simulink model "msdft_12_v2"  (R2013b)
settings: Solver=ode45  StartTime=0.0  StopTime=10.0  RelTol=1e-3
undefined symbols (not defined in the file or in its folder): msdft, sys_lib
libraries: xbsIndex_r4 x3195, casper_library_misc x152, casper_library_delays x42, dspsigops x32, xps_library x3
(part 4 of 33)

== system msdft_12_v2/corr3 ==
  addr : Inport
  data_in : Inport  Port=2
  we : Inport  Port=3
  calc_add : Subsystem  mask{data_width=128, addr_width=10, sample_rate=sample_rate}
      mask prompts: data_width "data width"; addr_width "address width"; sample_rate "sample rate"
  convert_addr : xbsIndex_r4/Convert  gui_display_data_type=Fixed-point  arith_type=Unsigned  n_bits=addr_width  bin_pt=0  float_type=Single  exp_bits=8  fraction_bits=24  quantization=Truncate  overflow=Wrap  en=off  latency=0  dbl_ovrd=off  pipeline=off  block_type=convert
      settings: xl_area=[0, 0, 0, 0, 0, 0, 0]
  convert_din1 : xbsIndex_r4/Convert  gui_display_data_type=Fixed-point  arith_type=Unsigned  n_bits=128  bin_pt=0  float_type=Single  exp_bits=8  fraction_bits=24  quantization=Truncate  overflow=Wrap  en=off  latency=0  dbl_ovrd=off  pipeline=off  block_type=convert
      settings: xl_area=[0, 0, 0, 0, 0, 0, 0]
  convert_we : xbsIndex_r4/Convert  gui_display_data_type=Fixed-point  arith_type=Unsigned  n_bits=1  bin_pt=0  float_type=Single  exp_bits=8  fraction_bits=24  quantization=Truncate  overflow=Wrap  en=off  latency=0  dbl_ovrd=off  pipeline=off  block_type=convert
      settings: xl_area=[0, 0, 0, 0, 0, 0, 0]
  mem : Subsystem
  msdft_12_v2_corr3_addr : xbsIndex_r4/Gateway Out  inherit_from_input=off  hdl_port=on  timing_constraint=None  locs_specified=off  LOCs={'A5','B9','A9','C1','A3','G6','E9','A6','A7','A8','B8','B1','B3','D9','B5','B4','B6','C2'}  UseAsDAC=off  DACChannel='1'  block_type=gatewayout
      settings: infoedit="Gateway out block.  Converts Xilinx fixed point inputs into ouputs of type Simulink integer, double, or fixed point.<P><P>Hardware notes:  In hardware these blocks become top level output ports or are discarded, depending on how they are configured."  xl_area=[0, 0, 0, 0, 0, 0, 0]  sginterface={'Nallatech'=>{'xdspkit'=>{'non_memory_mapped_port'=>'uprev_Shared_BRAM_addr'}},'Xilinx'=>{'jtaghwcosim'=>{'non_memory_mapped_port'=>'uprev_Shared_BRAM_addr'},'xdspkit'=>{'non_memory_mapped_port'=>'uprev_Shared_BRAM_addr'}}}
  msdft_12_v2_corr3_data_in : xbsIndex_r4/Gateway Out  inherit_from_input=off  hdl_port=on  timing_constraint=None  locs_specified=off  LOCs={'B21','B22','A22','B23','B19','C19','A20','A21','A23','B24','A24','A25','E18','D18','C18','B18'}  UseAsDAC=off  DACChannel='1'  block_type=gatewayout
      settings: infoedit="Gateway out block.  Converts Xilinx fixed point inputs into ouputs of type Simulink integer, double, or fixed point.<P><P>Hardware notes:  In hardware these blocks become top level output ports or are discarded, depending on how they are configured."  xl_area=[0, 0, 0, 0, 0, 0, 0]  sginterface={'Nallatech'=>{'xdspkit'=>{'non_memory_mapped_port'=>'uprev_Shared_BRAM_data_in'}},'Xilinx'=>{'jtaghwcosim'=>{'non_memory_mapped_port'=>'uprev_Shared_BRAM_data_in'},'xdspkit'=>{'non_memory_mapped_port'=>'uprev_Shared_BRAM_data_in'}}}
  msdft_12_v2_corr3_data_out : xbsIndex_r4/Gateway In  gui_display_data_type=Fixed-point  arith_type=Unsigned  n_bits=128  bin_pt=0  preci_type=Single  exp_width=8  frac_width=24  quantization=Truncate  overflow=Wrap  period=sample_rate  dbl_ovrd=off  timing_constraint=None  locs_specified=off  LOCs={}  UseAsADC=off  ADCChannel='1'  inherit_from_input=off  hdl_port=on  block_type=gatewayin
      settings: xl_area=[0, 0, 0, 0, 0, 0, 0]
  msdft_12_v2_corr3_we : xbsIndex_r4/Gateway Out  inherit_from_input=off  hdl_port=on  timing_constraint=None  locs_specified=off  LOCs={'A14'}  UseAsDAC=off  DACChannel='1'  block_type=gatewayout
      settings: infoedit="Gateway out block.  Converts Xilinx fixed point inputs into ouputs of type Simulink integer, double, or fixed point.<P><P>Hardware notes:  In hardware these blocks become top level output ports or are discarded, depending on how they are configured."  xl_area=[0, 0, 0, 0, 0, 0, 0]
  munge_in : Subsystem  AncestorBlock=casper_library_flow_control/munge  mask(munge){divisions=4, div_size=[32 32 32 32], order=[3  2  1  0], arith_type_out=Unsigned, bin_pt_out=0}
      mask prompts: divisions "Number of divisions"; div_size "Division size (bits)"; order "Division packing order"; arith_type_out "Output arithmetic type"; bin_pt_out "Output binary point"
      mask help: Splits an input bus into the specified number of divisions and then recombines them in the order specified (most significant division = 0,least = number divisions-1)
      mask init:
      | munge_init(gcb, ...
      |     'divisions', divisions, ...
      |     'div_size', div_size, ...
      |     'order', order, ...
      |     'arith_type_out', arith_type_out, ...
      |     'bin_pt_out', bin_pt_out);
      settings: AttributesFormatString=|
      | split:[32 32 32 32]
      | join:[3 2 1 0]
      | Unsigned [128,0]
      mask TypeOptions arith_type_out: Unsigned | Signed  (2's comp) | Floating-point
  munge_out : Subsystem  AncestorBlock=casper_library_flow_control/munge  mask(munge){divisions=4, div_size=[32 32 32 32], order=[3  2  1  0], arith_type_out=Unsigned, bin_pt_out=0}
      mask prompts: divisions "Number of divisions"; div_size "Division size (bits)"; order "Division packing order"; arith_type_out "Output arithmetic type"; bin_pt_out "Output binary point"
      mask help: Splits an input bus into the specified number of divisions and then recombines them in the order specified (most significant division = 0,least = number divisions-1)
      mask init:
      | munge_init(gcb, ...
      |     'divisions', divisions, ...
      |     'div_size', div_size, ...
      |     'order', order, ...
      |     'arith_type_out', arith_type_out, ...
      |     'bin_pt_out', bin_pt_out);
      settings: AttributesFormatString=|
      | split:[32 32 32 32]
      | join:[3 2 1 0]
      | Unsigned [128,0]
      mask TypeOptions arith_type_out: Unsigned | Signed  (2's comp) | Floating-point
  data_out : Outport
  wires:
  convert_addr/1 -> msdft_12_v2_corr3_addr/1
  convert_din1/1 -> msdft_12_v2_corr3_data_in/1
  data_in/1 -> munge_in/1(din)
  calc_add/1(out) -> convert_addr/1
  msdft_12_v2_corr3_we/1 -> mem/3(In3)
  msdft_12_v2_corr3_data_in/1 -> mem/2(In2)
  msdft_12_v2_corr3_addr/1 -> mem/1(In1)
  convert_we/1 -> msdft_12_v2_corr3_we/1
  msdft_12_v2_corr3_data_out/1 -> munge_out/1(din)
  mem/1(Out1) -> msdft_12_v2_corr3_data_out/1
  addr/1 -> calc_add/1(in)
  we/1 -> convert_we/1
  munge_out/1(dout) -> data_out/1
  munge_in/1(dout) -> convert_din1/1

== system msdft_12_v2/corr4 ==
  addr : Inport
  data_in : Inport  Port=2
  we : Inport  Port=3
  calc_add : Subsystem  mask{data_width=128, addr_width=10, sample_rate=sample_rate}
      mask prompts: data_width "data width"; addr_width "address width"; sample_rate "sample rate"
  convert_addr : xbsIndex_r4/Convert  gui_display_data_type=Fixed-point  arith_type=Unsigned  n_bits=addr_width  bin_pt=0  float_type=Single  exp_bits=8  fraction_bits=24  quantization=Truncate  overflow=Wrap  en=off  latency=0  dbl_ovrd=off  pipeline=off  block_type=convert
      settings: xl_area=[0, 0, 0, 0, 0, 0, 0]
  convert_din1 : xbsIndex_r4/Convert  gui_display_data_type=Fixed-point  arith_type=Unsigned  n_bits=128  bin_pt=0  float_type=Single  exp_bits=8  fraction_bits=24  quantization=Truncate  overflow=Wrap  en=off  latency=0  dbl_ovrd=off  pipeline=off  block_type=convert
      settings: xl_area=[0, 0, 0, 0, 0, 0, 0]
  convert_we : xbsIndex_r4/Convert  gui_display_data_type=Fixed-point  arith_type=Unsigned  n_bits=1  bin_pt=0  float_type=Single  exp_bits=8  fraction_bits=24  quantization=Truncate  overflow=Wrap  en=off  latency=0  dbl_ovrd=off  pipeline=off  block_type=convert
      settings: xl_area=[0, 0, 0, 0, 0, 0, 0]
  mem : Subsystem
  msdft_12_v2_corr4_addr : xbsIndex_r4/Gateway Out  inherit_from_input=off  hdl_port=on  timing_constraint=None  locs_specified=off  LOCs={'A5','B9','A9','C1','A3','G6','E9','A6','A7','A8','B8','B1','B3','D9','B5','B4','B6','C2'}  UseAsDAC=off  DACChannel='1'  block_type=gatewayout
      settings: infoedit="Gateway out block.  Converts Xilinx fixed point inputs into ouputs of type Simulink integer, double, or fixed point.<P><P>Hardware notes:  In hardware these blocks become top level output ports or are discarded, depending on how they are configured."  xl_area=[0, 0, 0, 0, 0, 0, 0]  sginterface={'Nallatech'=>{'xdspkit'=>{'non_memory_mapped_port'=>'uprev_Shared_BRAM_addr'}},'Xilinx'=>{'jtaghwcosim'=>{'non_memory_mapped_port'=>'uprev_Shared_BRAM_addr'},'xdspkit'=>{'non_memory_mapped_port'=>'uprev_Shared_BRAM_addr'}}}
  msdft_12_v2_corr4_data_in : xbsIndex_r4/Gateway Out  inherit_from_input=off  hdl_port=on  timing_constraint=None  locs_specified=off  LOCs={'B21','B22','A22','B23','B19','C19','A20','A21','A23','B24','A24','A25','E18','D18','C18','B18'}  UseAsDAC=off  DACChannel='1'  block_type=gatewayout
      settings: infoedit="Gateway out block.  Converts Xilinx fixed point inputs into ouputs of type Simulink integer, double, or fixed point.<P><P>Hardware notes:  In hardware these blocks become top level output ports or are discarded, depending on how they are configured."  xl_area=[0, 0, 0, 0, 0, 0, 0]  sginterface={'Nallatech'=>{'xdspkit'=>{'non_memory_mapped_port'=>'uprev_Shared_BRAM_data_in'}},'Xilinx'=>{'jtaghwcosim'=>{'non_memory_mapped_port'=>'uprev_Shared_BRAM_data_in'},'xdspkit'=>{'non_memory_mapped_port'=>'uprev_Shared_BRAM_data_in'}}}
  msdft_12_v2_corr4_data_out : xbsIndex_r4/Gateway In  gui_display_data_type=Fixed-point  arith_type=Unsigned  n_bits=128  bin_pt=0  preci_type=Single  exp_width=8  frac_width=24  quantization=Truncate  overflow=Wrap  period=sample_rate  dbl_ovrd=off  timing_constraint=None  locs_specified=off  LOCs={}  UseAsADC=off  ADCChannel='1'  inherit_from_input=off  hdl_port=on  block_type=gatewayin
      settings: xl_area=[0, 0, 0, 0, 0, 0, 0]
  msdft_12_v2_corr4_we : xbsIndex_r4/Gateway Out  inherit_from_input=off  hdl_port=on  timing_constraint=None  locs_specified=off  LOCs={'A14'}  UseAsDAC=off  DACChannel='1'  block_type=gatewayout
      settings: infoedit="Gateway out block.  Converts Xilinx fixed point inputs into ouputs of type Simulink integer, double, or fixed point.<P><P>Hardware notes:  In hardware these blocks become top level output ports or are discarded, depending on how they are configured."  xl_area=[0, 0, 0, 0, 0, 0, 0]
  munge_in : Subsystem  AncestorBlock=casper_library_flow_control/munge  mask(munge){divisions=4, div_size=[32 32 32 32], order=[3  2  1  0], arith_type_out=Unsigned, bin_pt_out=0}
      mask prompts: divisions "Number of divisions"; div_size "Division size (bits)"; order "Division packing order"; arith_type_out "Output arithmetic type"; bin_pt_out "Output binary point"
      mask help: Splits an input bus into the specified number of divisions and then recombines them in the order specified (most significant division = 0,least = number divisions-1)
      mask init:
      | munge_init(gcb, ...
      |     'divisions', divisions, ...
      |     'div_size', div_size, ...
      |     'order', order, ...
      |     'arith_type_out', arith_type_out, ...
      |     'bin_pt_out', bin_pt_out);
      settings: AttributesFormatString=|
      | split:[32 32 32 32]
      | join:[3 2 1 0]
      | Unsigned [128,0]
      mask TypeOptions arith_type_out: Unsigned | Signed  (2's comp) | Floating-point
  munge_out : Subsystem  AncestorBlock=casper_library_flow_control/munge  mask(munge){divisions=4, div_size=[32 32 32 32], order=[3  2  1  0], arith_type_out=Unsigned, bin_pt_out=0}
      mask prompts: divisions "Number of divisions"; div_size "Division size (bits)"; order "Division packing order"; arith_type_out "Output arithmetic type"; bin_pt_out "Output binary point"
      mask help: Splits an input bus into the specified number of divisions and then recombines them in the order specified (most significant division = 0,least = number divisions-1)
      mask init:
      | munge_init(gcb, ...
      |     'divisions', divisions, ...
      |     'div_size', div_size, ...
      |     'order', order, ...
      |     'arith_type_out', arith_type_out, ...
      |     'bin_pt_out', bin_pt_out);
      settings: AttributesFormatString=|
      | split:[32 32 32 32]
      | join:[3 2 1 0]
      | Unsigned [128,0]
      mask TypeOptions arith_type_out: Unsigned | Signed  (2's comp) | Floating-point
  data_out : Outport
  wires:
  convert_addr/1 -> msdft_12_v2_corr4_addr/1
  convert_din1/1 -> msdft_12_v2_corr4_data_in/1
  data_in/1 -> munge_in/1(din)
  calc_add/1(out) -> convert_addr/1
  msdft_12_v2_corr4_we/1 -> mem/3(In3)
  msdft_12_v2_corr4_data_in/1 -> mem/2(In2)
  msdft_12_v2_corr4_addr/1 -> mem/1(In1)
  convert_we/1 -> msdft_12_v2_corr4_we/1
  msdft_12_v2_corr4_data_out/1 -> munge_out/1(din)
  mem/1(Out1) -> msdft_12_v2_corr4_data_out/1
  addr/1 -> calc_add/1(in)
  we/1 -> convert_we/1
  munge_out/1(dout) -> data_out/1
  munge_in/1(dout) -> convert_din1/1

== system msdft_12_v2/corr5 ==
  addr : Inport
  data_in : Inport  Port=2
  we : Inport  Port=3
  calc_add : Subsystem  mask{data_width=128, addr_width=10, sample_rate=sample_rate}
      mask prompts: data_width "data width"; addr_width "address width"; sample_rate "sample rate"
  convert_addr : xbsIndex_r4/Convert  gui_display_data_type=Fixed-point  arith_type=Unsigned  n_bits=addr_width  bin_pt=0  float_type=Single  exp_bits=8  fraction_bits=24  quantization=Truncate  overflow=Wrap  en=off  latency=0  dbl_ovrd=off  pipeline=off  block_type=convert
      settings: xl_area=[0, 0, 0, 0, 0, 0, 0]
  convert_din1 : xbsIndex_r4/Convert  gui_display_data_type=Fixed-point  arith_type=Unsigned  n_bits=128  bin_pt=0  float_type=Single  exp_bits=8  fraction_bits=24  quantization=Truncate  overflow=Wrap  en=off  latency=0  dbl_ovrd=off  pipeline=off  block_type=convert
      settings: xl_area=[0, 0, 0, 0, 0, 0, 0]
  convert_we : xbsIndex_r4/Convert  gui_display_data_type=Fixed-point  arith_type=Unsigned  n_bits=1  bin_pt=0  float_type=Single  exp_bits=8  fraction_bits=24  quantization=Truncate  overflow=Wrap  en=off  latency=0  dbl_ovrd=off  pipeline=off  block_type=convert
      settings: xl_area=[0, 0, 0, 0, 0, 0, 0]
  mem : Subsystem
  msdft_12_v2_corr5_addr : xbsIndex_r4/Gateway Out  inherit_from_input=off  hdl_port=on  timing_constraint=None  locs_specified=off  LOCs={'A5','B9','A9','C1','A3','G6','E9','A6','A7','A8','B8','B1','B3','D9','B5','B4','B6','C2'}  UseAsDAC=off  DACChannel='1'  block_type=gatewayout
      settings: infoedit="Gateway out block.  Converts Xilinx fixed point inputs into ouputs of type Simulink integer, double, or fixed point.<P><P>Hardware notes:  In hardware these blocks become top level output ports or are discarded, depending on how they are configured."  xl_area=[0, 0, 0, 0, 0, 0, 0]  sginterface={'Nallatech'=>{'xdspkit'=>{'non_memory_mapped_port'=>'uprev_Shared_BRAM_addr'}},'Xilinx'=>{'jtaghwcosim'=>{'non_memory_mapped_port'=>'uprev_Shared_BRAM_addr'},'xdspkit'=>{'non_memory_mapped_port'=>'uprev_Shared_BRAM_addr'}}}
  msdft_12_v2_corr5_data_in : xbsIndex_r4/Gateway Out  inherit_from_input=off  hdl_port=on  timing_constraint=None  locs_specified=off  LOCs={'B21','B22','A22','B23','B19','C19','A20','A21','A23','B24','A24','A25','E18','D18','C18','B18'}  UseAsDAC=off  DACChannel='1'  block_type=gatewayout
      settings: infoedit="Gateway out block.  Converts Xilinx fixed point inputs into ouputs of type Simulink integer, double, or fixed point.<P><P>Hardware notes:  In hardware these blocks become top level output ports or are discarded, depending on how they are configured."  xl_area=[0, 0, 0, 0, 0, 0, 0]  sginterface={'Nallatech'=>{'xdspkit'=>{'non_memory_mapped_port'=>'uprev_Shared_BRAM_data_in'}},'Xilinx'=>{'jtaghwcosim'=>{'non_memory_mapped_port'=>'uprev_Shared_BRAM_data_in'},'xdspkit'=>{'non_memory_mapped_port'=>'uprev_Shared_BRAM_data_in'}}}
  msdft_12_v2_corr5_data_out : xbsIndex_r4/Gateway In  gui_display_data_type=Fixed-point  arith_type=Unsigned  n_bits=128  bin_pt=0  preci_type=Single  exp_width=8  frac_width=24  quantization=Truncate  overflow=Wrap  period=sample_rate  dbl_ovrd=off  timing_constraint=None  locs_specified=off  LOCs={}  UseAsADC=off  ADCChannel='1'  inherit_from_input=off  hdl_port=on  block_type=gatewayin
      settings: xl_area=[0, 0, 0, 0, 0, 0, 0]
  msdft_12_v2_corr5_we : xbsIndex_r4/Gateway Out  inherit_from_input=off  hdl_port=on  timing_constraint=None  locs_specified=off  LOCs={'A14'}  UseAsDAC=off  DACChannel='1'  block_type=gatewayout
      settings: infoedit="Gateway out block.  Converts Xilinx fixed point inputs into ouputs of type Simulink integer, double, or fixed point.<P><P>Hardware notes:  In hardware these blocks become top level output ports or are discarded, depending on how they are configured."  xl_area=[0, 0, 0, 0, 0, 0, 0]
  munge_in : Subsystem  AncestorBlock=casper_library_flow_control/munge  mask(munge){divisions=4, div_size=[32 32 32 32], order=[3  2  1  0], arith_type_out=Unsigned, bin_pt_out=0}
      mask prompts: divisions "Number of divisions"; div_size "Division size (bits)"; order "Division packing order"; arith_type_out "Output arithmetic type"; bin_pt_out "Output binary point"
      mask help: Splits an input bus into the specified number of divisions and then recombines them in the order specified (most significant division = 0,least = number divisions-1)
      mask init:
      | munge_init(gcb, ...
      |     'divisions', divisions, ...
      |     'div_size', div_size, ...
      |     'order', order, ...
      |     'arith_type_out', arith_type_out, ...
      |     'bin_pt_out', bin_pt_out);
      settings: AttributesFormatString=|
      | split:[32 32 32 32]
      | join:[3 2 1 0]
      | Unsigned [128,0]
      mask TypeOptions arith_type_out: Unsigned | Signed  (2's comp) | Floating-point
  munge_out : Subsystem  AncestorBlock=casper_library_flow_control/munge  mask(munge){divisions=4, div_size=[32 32 32 32], order=[3  2  1  0], arith_type_out=Unsigned, bin_pt_out=0}
      mask prompts: divisions "Number of divisions"; div_size "Division size (bits)"; order "Division packing order"; arith_type_out "Output arithmetic type"; bin_pt_out "Output binary point"
      mask help: Splits an input bus into the specified number of divisions and then recombines them in the order specified (most significant division = 0,least = number divisions-1)
      mask init:
      | munge_init(gcb, ...
      |     'divisions', divisions, ...
      |     'div_size', div_size, ...
      |     'order', order, ...
      |     'arith_type_out', arith_type_out, ...
      |     'bin_pt_out', bin_pt_out);
      settings: AttributesFormatString=|
      | split:[32 32 32 32]
      | join:[3 2 1 0]
      | Unsigned [128,0]
      mask TypeOptions arith_type_out: Unsigned | Signed  (2's comp) | Floating-point
  data_out : Outport
  wires:
  convert_addr/1 -> msdft_12_v2_corr5_addr/1
  convert_din1/1 -> msdft_12_v2_corr5_data_in/1
  data_in/1 -> munge_in/1(din)
  calc_add/1(out) -> convert_addr/1
  msdft_12_v2_corr5_we/1 -> mem/3(In3)
  msdft_12_v2_corr5_data_in/1 -> mem/2(In2)
  msdft_12_v2_corr5_addr/1 -> mem/1(In1)
  convert_we/1 -> msdft_12_v2_corr5_we/1
  msdft_12_v2_corr5_data_out/1 -> munge_out/1(din)
  mem/1(Out1) -> msdft_12_v2_corr5_data_out/1
  addr/1 -> calc_add/1(in)
  we/1 -> convert_we/1
  munge_out/1(dout) -> data_out/1
  munge_in/1(dout) -> convert_din1/1

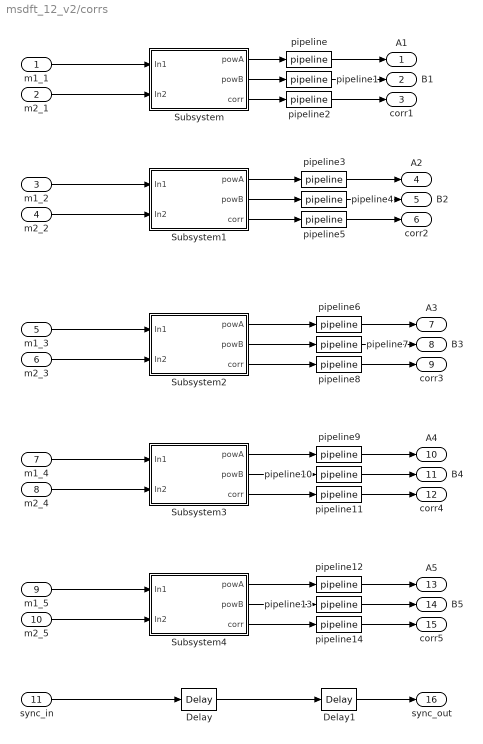
== system msdft_12_v2/corrs ==
  m1_1 : Inport
  m2_1 : Inport  Port=2
  m1_2 : Inport  Port=3
  m2_2 : Inport  Port=4
  m1_3 : Inport  Port=5
  m2_3 : Inport  Port=6
  m1_4 : Inport  Port=7
  m2_4 : Inport  Port=8
  m1_5 : Inport  Port=9
  m2_5 : Inport  Port=10
  sync_in : Inport  Port=11
  Delay : xbsIndex_r4/Delay  rst=off  infoeditControl=Selection of Reset will increase slice count due to use of real FFs and instead of SRLs  en=off  latency=10  dbl_ovrd=off  reg_retiming=off  block_type=delay
  Delay1 : xbsIndex_r4/Delay  rst=off  infoeditControl=Selection of Reset will increase slice count due to use of real FFs and instead of SRLs  en=off  latency=3  dbl_ovrd=off  reg_retiming=off  block_type=delay
  Subsystem : Subsystem
  Subsystem1 : Subsystem
  Subsystem2 : Subsystem
  Subsystem3 : Subsystem
  Subsystem4 : Subsystem
  pipeline{,1..14} (15 alike) : casper_library_delays/pipeline  latency=3
      settings: AttributesFormatString=Latency = %<latency>
  A1 : Outport
  B1 : Outport  Port=2
  corr1 : Outport  Port=3
  A2 : Outport  Port=4
  B2 : Outport  Port=5
  corr2 : Outport  Port=6
  A3 : Outport  Port=7
  B3 : Outport  Port=8
  corr3 : Outport  Port=9
  A4 : Outport  Port=10
  B4 : Outport  Port=11
  corr4 : Outport  Port=12
  A5 : Outport  Port=13
  B5 : Outport  Port=14
  corr5 : Outport  Port=15
  sync_out : Outport  Port=16
  wires:
  m1_1/1 -> Subsystem/1(In1)
  m2_1/1 -> Subsystem/2(In2)
  m1_2/1 -> Subsystem1/1(In1)
  m2_2/1 -> Subsystem1/2(In2)
  m1_3/1 -> Subsystem2/1(In1)
  m2_3/1 -> Subsystem2/2(In2)
  m1_4/1 -> Subsystem3/1(In1)
  m2_4/1 -> Subsystem3/2(In2)
  m1_5/1 -> Subsystem4/1(In1)
  m2_5/1 -> Subsystem4/2(In2)
  Subsystem/1(powA) -> pipeline/1
  Subsystem/2(powB) -> pipeline1/1
  Subsystem/3(corr) -> pipeline2/1
  pipeline/1 -> A1/1
  pipeline1/1 -> B1/1
  pipeline2/1 -> corr1/1
  pipeline3/1 -> A2/1
  pipeline4/1 -> B2/1
  pipeline5/1 -> corr2/1
  Subsystem1/1(powA) -> pipeline3/1
  Subsystem1/2(powB) -> pipeline4/1
  Subsystem1/3(corr) -> pipeline5/1
  pipeline6/1 -> A3/1
  pipeline7/1 -> B3/1
  pipeline8/1 -> corr3/1
  Subsystem2/1(powA) -> pipeline6/1
  Subsystem2/2(powB) -> pipeline7/1
  Subsystem2/3(corr) -> pipeline8/1
  pipeline9/1 -> A4/1
  pipeline10/1 -> B4/1
  pipeline11/1 -> corr4/1
  Subsystem3/1(powA) -> pipeline9/1
  Subsystem3/2(powB) -> pipeline10/1
  Subsystem3/3(corr) -> pipeline11/1
  pipeline12/1 -> A5/1
  pipeline13/1 -> B5/1
  pipeline14/1 -> corr5/1
  Subsystem4/1(powA) -> pipeline12/1
  Subsystem4/2(powB) -> pipeline13/1
  Subsystem4/3(corr) -> pipeline14/1
  sync_in/1 -> Delay/1
  Delay/1 -> Delay1/1
  Delay1/1 -> sync_out/1

== system msdft_12_v2/mem_addr ==
  sim_1 : Inport
  io_delay : xbsIndex_r4/Delay  rst=off  infoeditControl=Selection of Reset will increase slice count due to use of real FFs and instead of SRLs  en=off  latency=0  dbl_ovrd=off  reg_retiming=on  block_type=delay
  msdft_12_v2_mem_addr_user_data_out : xbsIndex_r4/Gateway In  gui_display_data_type=Fixed-point  arith_type=Unsigned  n_bits=32  bin_pt=0  preci_type=Single  exp_width=8  frac_width=24  quantization="Round  (unbiased: +/- Inf)"  overflow=Saturate  period=1  dbl_ovrd=off  timing_constraint=None  locs_specified=off  LOCs={}  UseAsADC=off  ADCChannel='1'  inherit_from_input=off  hdl_port=on  block_type=gatewayin
  reint1 : xbsIndex_r4/Reinterpret  force_arith_type=on  arith_type=Unsigned  force_bin_pt=on  bin_pt=0  block_type=reinterpret
  slice_reg : xbsIndex_r4/Slice  nbits=32  boolean_output=off  mode=Lower Bit Location + Width  bit1=0  base1=MSB of Input  bit0=0  base0=LSB of Input  dbl_ovrd=off  block_type=slice
  in_reg : Outport
  wires:
  msdft_12_v2_mem_addr_user_data_out/1 -> io_delay/1
  sim_1/1 -> msdft_12_v2_mem_addr_user_data_out/1
  io_delay/1 -> slice_reg/1
  slice_reg/1 -> reint1/1
  reint1/1 -> in_reg/1

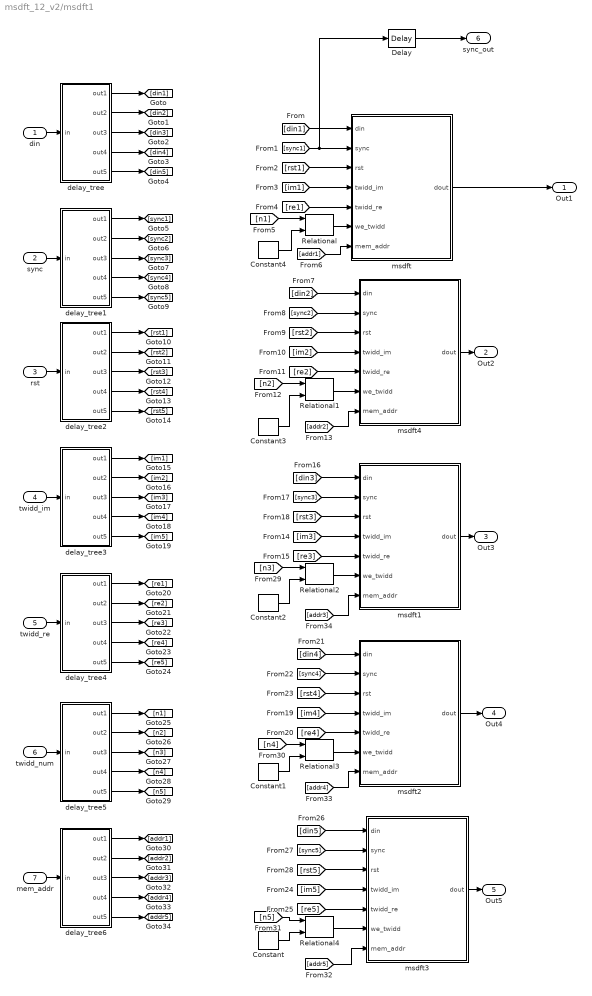
== system msdft_12_v2/msdft1 ==
  din : Inport
  "sync " : Inport  Port=2
  rst : Inport  Port=3
  twidd_im : Inport  Port=4
  twidd_re : Inport  Port=5
  twidd_num : Inport  Port=6
  mem_addr : Inport  Port=7
  Constant : xbsIndex_r4/Constant  const=5  gui_display_data_type=Fixed-point  arith_type=Unsigned  n_bits=16  bin_pt=0  preci_type=Single  exp_width=8  frac_width=24  explicit_period=on  period=1  equ=P=C  opselect=C  inp2=PCIN>>17  opr=+  inp1=P  carry=CIN  dbl_ovrd=off  block_type=constant
  Constant1 : xbsIndex_r4/Constant  const=4  gui_display_data_type=Fixed-point  arith_type=Unsigned  n_bits=16  bin_pt=0  preci_type=Single  exp_width=8  frac_width=24  explicit_period=on  period=1  equ=P=C  opselect=C  inp2=PCIN>>17  opr=+  inp1=P  carry=CIN  dbl_ovrd=off  block_type=constant
  Constant2 : xbsIndex_r4/Constant  const=3  gui_display_data_type=Fixed-point  arith_type=Unsigned  n_bits=16  bin_pt=0  preci_type=Single  exp_width=8  frac_width=24  explicit_period=on  period=1  equ=P=C  opselect=C  inp2=PCIN>>17  opr=+  inp1=P  carry=CIN  dbl_ovrd=off  block_type=constant
  Constant3 : xbsIndex_r4/Constant  const=2  gui_display_data_type=Fixed-point  arith_type=Unsigned  n_bits=16  bin_pt=0  preci_type=Single  exp_width=8  frac_width=24  explicit_period=on  period=1  equ=P=C  opselect=C  inp2=PCIN>>17  opr=+  inp1=P  carry=CIN  dbl_ovrd=off  block_type=constant
  Constant4 : xbsIndex_r4/Constant  const=1  gui_display_data_type=Fixed-point  arith_type=Unsigned  n_bits=16  bin_pt=0  preci_type=Single  exp_width=8  frac_width=24  explicit_period=on  period=1  equ=P=C  opselect=C  inp2=PCIN>>17  opr=+  inp1=P  carry=CIN  dbl_ovrd=off  block_type=constant
  Delay : xbsIndex_r4/Delay  rst=off  infoeditControl=Selection of Reset will increase slice count due to use of real FFs and instead of SRLs  en=off  latency=2^12+10  dbl_ovrd=off  reg_retiming=off  block_type=delay
  Relational{,1..4} (5 alike) : xbsIndex_r4/Relational  mode=a=b  en=off  latency=0  dbl_ovrd=off  block_type=relational
  delay_tree : Subsystem  AncestorBlock=casper_library_delays/delay_tree  mask(delay_tree){fanout=5, bfac=2}
      mask prompts: bfac "Branching factor"
      mask help: A tree of delays.
      mask init:
      | delay_tree_init(gcb, ...
      |     'fanout', fanout, ...
      |     'bfac', bfac);
      settings: AttributesFormatString=delay=4
  delay_tree1 : Subsystem  AncestorBlock=casper_library_delays/delay_tree  mask(delay_tree){fanout=5, bfac=2}
      mask prompts: bfac "Branching factor"
      mask help: A tree of delays.
      mask init:
      | delay_tree_init(gcb, ...
      |     'fanout', fanout, ...
      |     'bfac', bfac);
      settings: AttributesFormatString=delay=4
  delay_tree2 : Subsystem  AncestorBlock=casper_library_delays/delay_tree  mask(delay_tree){fanout=5, bfac=2}
      mask prompts: bfac "Branching factor"
      mask help: A tree of delays.
      mask init:
      | delay_tree_init(gcb, ...
      |     'fanout', fanout, ...
      |     'bfac', bfac);
      settings: AttributesFormatString=delay=4
  delay_tree3 : Subsystem  AncestorBlock=casper_library_delays/delay_tree  mask(delay_tree){fanout=5, bfac=2}
      mask prompts: bfac "Branching factor"
      mask help: A tree of delays.
      mask init:
      | delay_tree_init(gcb, ...
      |     'fanout', fanout, ...
      |     'bfac', bfac);
      settings: AttributesFormatString=delay=4
  delay_tree4 : Subsystem  AncestorBlock=casper_library_delays/delay_tree  mask(delay_tree){fanout=5, bfac=2}
      mask prompts: bfac "Branching factor"
      mask help: A tree of delays.
      mask init:
      | delay_tree_init(gcb, ...
      |     'fanout', fanout, ...
      |     'bfac', bfac);
      settings: AttributesFormatString=delay=4
  delay_tree5 : Subsystem  AncestorBlock=casper_library_delays/delay_tree  mask(delay_tree){fanout=5, bfac=2}
      mask prompts: bfac "Branching factor"
      mask help: A tree of delays.
      mask init:
      | delay_tree_init(gcb, ...
      |     'fanout', fanout, ...
      |     'bfac', bfac);
      settings: AttributesFormatString=delay=4
  delay_tree6 : Subsystem  AncestorBlock=casper_library_delays/delay_tree  mask(delay_tree){fanout=5, bfac=2}
      mask prompts: bfac "Branching factor"
      mask help: A tree of delays.
      mask init:
      | delay_tree_init(gcb, ...
      |     'fanout', fanout, ...
      |     'bfac', bfac);
      settings: AttributesFormatString=delay=4
  msdft : Subsystem  AncestorBlock=sys_lib/msdft  mask{in_bit=8, N=12, init_twidd=1397, twidd_bit=16, out_bit=25}
      mask prompts: in_bit "input bitwidth"; N "dft size (2^?)"; init_twidd "init twiddle factor"; twidd_bit "bitsize twiddle factor"; out_bit "output bitwidth"
  msdft1 : Subsystem  AncestorBlock=sys_lib/msdft  mask{in_bit=8, N=12, init_twidd=1399, twidd_bit=16, out_bit=25}
      mask prompts: in_bit "input bitwidth"; N "dft size (2^?)"; init_twidd "init twiddle factor"; twidd_bit "bitsize twiddle factor"; out_bit "output bitwidth"
  msdft2 : Subsystem  AncestorBlock=sys_lib/msdft  mask{in_bit=8, N=12, init_twidd=1400, twidd_bit=16, out_bit=25}
      mask prompts: in_bit "input bitwidth"; N "dft size (2^?)"; init_twidd "init twiddle factor"; twidd_bit "bitsize twiddle factor"; out_bit "output bitwidth"
  msdft3 : Subsystem  AncestorBlock=sys_lib/msdft  mask{in_bit=8, N=12, init_twidd=1401, twidd_bit=16, out_bit=25}
      mask prompts: in_bit "input bitwidth"; N "dft size (2^?)"; init_twidd "init twiddle factor"; twidd_bit "bitsize twiddle factor"; out_bit "output bitwidth"
  msdft4 : Subsystem  AncestorBlock=sys_lib/msdft  mask{in_bit=8, N=12, init_twidd=1398, twidd_bit=16, out_bit=25}
      mask prompts: in_bit "input bitwidth"; N "dft size (2^?)"; init_twidd "init twiddle factor"; twidd_bit "bitsize twiddle factor"; out_bit "output bitwidth"
  Out1 : Outport
  Out2 : Outport  Port=2
  Out3 : Outport  Port=3
  Out4 : Outport  Port=4
  Out5 : Outport  Port=5
  sync_out : Outport  Port=6
  wires:
  Constant3/1 -> Relational1/2
  [addr3] -> msdft1/7(mem_addr)
  [din5] -> msdft3/1(din)
  delay_tree6/1(out1) -> [addr1]
  Constant4/1 -> Relational/2
  msdft1/1(dout) -> Out3/1
  delay_tree6/3(out3) -> [addr3]
  [rst5] -> msdft3/3(rst)
  delay_tree5/4(out4) -> [n4]
  delay_tree5/5(out5) -> [n5]
  Constant2/1 -> Relational2/2
  delay_tree2/3(out3) -> [rst3]
  delay_tree4/1(out1) -> [re1]
  delay_tree3/4(out4) -> [im4]
  [rst1] -> msdft/3(rst)
  [re3] -> msdft1/5(twidd_re)
  [n3] -> Relational2/1
  delay_tree6/2(out2) -> [addr2]
  "sync "/1 -> delay_tree1/1(in)
  [addr5] -> msdft3/7(mem_addr)
  delay_tree/2(out2) -> [din2]
  delay_tree1/2(out2) -> [sync2]
  twidd_re/1 -> delay_tree4/1(in)
  delay_tree/3(out3) -> [din3]
  [din2] -> msdft4/1(din)
  Relational4/1 -> msdft3/6(we_twidd)
  [re5] -> msdft3/5(twidd_re)
  Relational1/1 -> msdft4/6(we_twidd)
  [re4] -> msdft2/5(twidd_re)
  delay_tree2/5(out5) -> [rst5]
  [sync4] -> msdft2/2(sync)
  delay_tree2/2(out2) -> [rst2]
  delay_tree/1(out1) -> [din1]
  [re2] -> msdft4/5(twidd_re)
  [sync1] -> Delay/1, msdft/2(sync)
  delay_tree4/3(out3) -> [re3]
  din/1 -> delay_tree/1(in)
  [sync5] -> msdft3/2(sync)
  [din4] -> msdft2/1(din)
  delay_tree3/1(out1) -> [im1]
  delay_tree1/4(out4) -> [sync4]
  delay_tree4/2(out2) -> [re2]
  [n5] -> Relational4/1
  delay_tree5/2(out2) -> [n2]
  [sync3] -> msdft1/2(sync)
  delay_tree1/5(out5) -> [sync5]
  delay_tree5/3(out3) -> [n3]
  [addr2] -> msdft4/7(mem_addr)
  [rst4] -> msdft2/3(rst)
  twidd_num/1 -> delay_tree5/1(in)
  Constant1/1 -> Relational3/2
  delay_tree5/1(out1) -> [n1]
  [din3] -> msdft1/1(din)
  rst/1 -> delay_tree2/1(in)
  msdft2/1(dout) -> Out4/1
  [addr1] -> msdft/7(mem_addr)
  [addr4] -> msdft2/7(mem_addr)
  delay_tree3/2(out2) -> [im2]
  delay_tree2/1(out1) -> [rst1]
  [im5] -> msdft3/4(twidd_im)
  delay_tree6/4(out4) -> [addr4]
  [n4] -> Relational3/1
  twidd_im/1 -> delay_tree3/1(in)
  [im1] -> msdft/4(twidd_im)
  delay_tree3/5(out5) -> [im5]
  msdft/1(dout) -> Out1/1
  [im4] -> msdft2/4(twidd_im)
  Relational/1 -> msdft/6(we_twidd)
  delay_tree3/3(out3) -> [im3]
  delay_tree2/4(out4) -> [rst4]
  [n2] -> Relational1/1
  [din1] -> msdft/1(din)
  delay_tree1/1(out1) -> [sync1]
  [im3] -> msdft1/4(twidd_im)
  Constant/1 -> Relational4/2
  delay_tree4/4(out4) -> [re4]
  [im2] -> msdft4/4(twidd_im)
  delay_tree4/5(out5) -> [re5]
  delay_tree6/5(out5) -> [addr5]
  delay_tree1/3(out3) -> [sync3]
  [rst3] -> msdft1/3(rst)
  [rst2] -> msdft4/3(rst)
  [n1] -> Relational/1
  Relational2/1 -> msdft1/6(we_twidd)
  [sync2] -> msdft4/2(sync)
  [re1] -> msdft/5(twidd_re)
  delay_tree/4(out4) -> [din4]
  Relational3/1 -> msdft2/6(we_twidd)
  mem_addr/1 -> delay_tree6/1(in)
  delay_tree/5(out5) -> [din5]
  Delay/1 -> sync_out/1
  msdft4/1(dout) -> Out2/1
  msdft3/1(dout) -> Out5/1

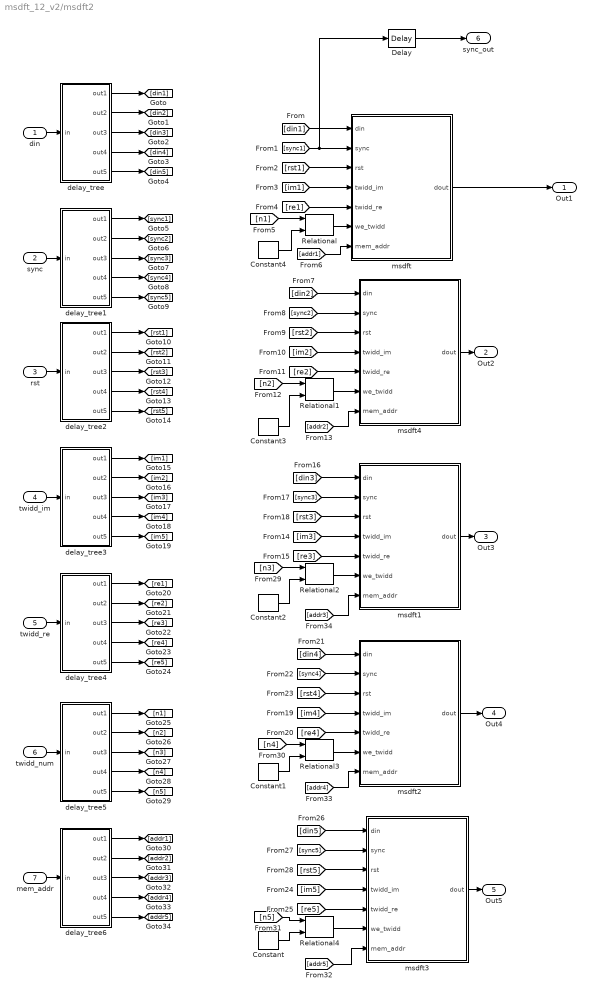
== system msdft_12_v2/msdft2 ==
  din : Inport
  "sync " : Inport  Port=2
  rst : Inport  Port=3
  twidd_im : Inport  Port=4
  twidd_re : Inport  Port=5
  twidd_num : Inport  Port=6
  mem_addr : Inport  Port=7
  Constant : xbsIndex_r4/Constant  const=5  gui_display_data_type=Fixed-point  arith_type=Unsigned  n_bits=16  bin_pt=0  preci_type=Single  exp_width=8  frac_width=24  explicit_period=on  period=1  equ=P=C  opselect=C  inp2=PCIN>>17  opr=+  inp1=P  carry=CIN  dbl_ovrd=off  block_type=constant
  Constant1 : xbsIndex_r4/Constant  const=4  gui_display_data_type=Fixed-point  arith_type=Unsigned  n_bits=16  bin_pt=0  preci_type=Single  exp_width=8  frac_width=24  explicit_period=on  period=1  equ=P=C  opselect=C  inp2=PCIN>>17  opr=+  inp1=P  carry=CIN  dbl_ovrd=off  block_type=constant
  Constant2 : xbsIndex_r4/Constant  const=3  gui_display_data_type=Fixed-point  arith_type=Unsigned  n_bits=16  bin_pt=0  preci_type=Single  exp_width=8  frac_width=24  explicit_period=on  period=1  equ=P=C  opselect=C  inp2=PCIN>>17  opr=+  inp1=P  carry=CIN  dbl_ovrd=off  block_type=constant
  Constant3 : xbsIndex_r4/Constant  const=2  gui_display_data_type=Fixed-point  arith_type=Unsigned  n_bits=16  bin_pt=0  preci_type=Single  exp_width=8  frac_width=24  explicit_period=on  period=1  equ=P=C  opselect=C  inp2=PCIN>>17  opr=+  inp1=P  carry=CIN  dbl_ovrd=off  block_type=constant
  Constant4 : xbsIndex_r4/Constant  const=1  gui_display_data_type=Fixed-point  arith_type=Unsigned  n_bits=16  bin_pt=0  preci_type=Single  exp_width=8  frac_width=24  explicit_period=on  period=1  equ=P=C  opselect=C  inp2=PCIN>>17  opr=+  inp1=P  carry=CIN  dbl_ovrd=off  block_type=constant
  Delay : xbsIndex_r4/Delay  rst=off  infoeditControl=Selection of Reset will increase slice count due to use of real FFs and instead of SRLs  en=off  latency=2^12+10  dbl_ovrd=off  reg_retiming=off  block_type=delay
  Relational{,1..4} (5 alike) : xbsIndex_r4/Relational  mode=a=b  en=off  latency=0  dbl_ovrd=off  block_type=relational
  delay_tree : Subsystem  AncestorBlock=casper_library_delays/delay_tree  mask(delay_tree){fanout=5, bfac=2}
      mask prompts: bfac "Branching factor"
      mask help: A tree of delays.
      mask init:
      | delay_tree_init(gcb, ...
      |     'fanout', fanout, ...
      |     'bfac', bfac);
      settings: AttributesFormatString=delay=4
  delay_tree1 : Subsystem  AncestorBlock=casper_library_delays/delay_tree  mask(delay_tree){fanout=5, bfac=2}
      mask prompts: bfac "Branching factor"
      mask help: A tree of delays.
      mask init:
      | delay_tree_init(gcb, ...
      |     'fanout', fanout, ...
      |     'bfac', bfac);
      settings: AttributesFormatString=delay=4
  delay_tree2 : Subsystem  AncestorBlock=casper_library_delays/delay_tree  mask(delay_tree){fanout=5, bfac=2}
      mask prompts: bfac "Branching factor"
      mask help: A tree of delays.
      mask init:
      | delay_tree_init(gcb, ...
      |     'fanout', fanout, ...
      |     'bfac', bfac);
      settings: AttributesFormatString=delay=4
  delay_tree3 : Subsystem  AncestorBlock=casper_library_delays/delay_tree  mask(delay_tree){fanout=5, bfac=2}
      mask prompts: bfac "Branching factor"
      mask help: A tree of delays.
      mask init:
      | delay_tree_init(gcb, ...
      |     'fanout', fanout, ...
      |     'bfac', bfac);
      settings: AttributesFormatString=delay=4
  delay_tree4 : Subsystem  AncestorBlock=casper_library_delays/delay_tree  mask(delay_tree){fanout=5, bfac=2}
      mask prompts: bfac "Branching factor"
      mask help: A tree of delays.
      mask init:
      | delay_tree_init(gcb, ...
      |     'fanout', fanout, ...
      |     'bfac', bfac);
      settings: AttributesFormatString=delay=4
  delay_tree5 : Subsystem  AncestorBlock=casper_library_delays/delay_tree  mask(delay_tree){fanout=5, bfac=2}
      mask prompts: bfac "Branching factor"
      mask help: A tree of delays.
      mask init:
      | delay_tree_init(gcb, ...
      |     'fanout', fanout, ...
      |     'bfac', bfac);
      settings: AttributesFormatString=delay=4
  delay_tree6 : Subsystem  AncestorBlock=casper_library_delays/delay_tree  mask(delay_tree){fanout=5, bfac=2}
      mask prompts: bfac "Branching factor"
      mask help: A tree of delays.
      mask init:
      | delay_tree_init(gcb, ...
      |     'fanout', fanout, ...
      |     'bfac', bfac);
      settings: AttributesFormatString=delay=4
  msdft : Subsystem  AncestorBlock=sys_lib/msdft  mask{in_bit=8, N=12, init_twidd=1397, twidd_bit=16, out_bit=25}
      mask prompts: in_bit "input bitwidth"; N "dft size (2^?)"; init_twidd "init twiddle factor"; twidd_bit "bitsize twiddle factor"; out_bit "output bitwidth"
  msdft1 : Subsystem  AncestorBlock=sys_lib/msdft  mask{in_bit=8, N=12, init_twidd=1399, twidd_bit=16, out_bit=25}
      mask prompts: in_bit "input bitwidth"; N "dft size (2^?)"; init_twidd "init twiddle factor"; twidd_bit "bitsize twiddle factor"; out_bit "output bitwidth"
  msdft2 : Subsystem  AncestorBlock=sys_lib/msdft  mask{in_bit=8, N=12, init_twidd=1400, twidd_bit=16, out_bit=25}
      mask prompts: in_bit "input bitwidth"; N "dft size (2^?)"; init_twidd "init twiddle factor"; twidd_bit "bitsize twiddle factor"; out_bit "output bitwidth"
  msdft3 : Subsystem  AncestorBlock=sys_lib/msdft  mask{in_bit=8, N=12, init_twidd=1401, twidd_bit=16, out_bit=25}
      mask prompts: in_bit "input bitwidth"; N "dft size (2^?)"; init_twidd "init twiddle factor"; twidd_bit "bitsize twiddle factor"; out_bit "output bitwidth"
  msdft4 : Subsystem  AncestorBlock=sys_lib/msdft  mask{in_bit=8, N=12, init_twidd=1398, twidd_bit=16, out_bit=25}
      mask prompts: in_bit "input bitwidth"; N "dft size (2^?)"; init_twidd "init twiddle factor"; twidd_bit "bitsize twiddle factor"; out_bit "output bitwidth"
  Out1 : Outport
  Out2 : Outport  Port=2
  Out3 : Outport  Port=3
  Out4 : Outport  Port=4
  Out5 : Outport  Port=5
  sync_out : Outport  Port=6
  wires:
  Constant3/1 -> Relational1/2
  [addr3] -> msdft1/7(mem_addr)
  [din5] -> msdft3/1(din)
  delay_tree6/1(out1) -> [addr1]
  Constant4/1 -> Relational/2
  msdft1/1(dout) -> Out3/1
  delay_tree6/3(out3) -> [addr3]
  [rst5] -> msdft3/3(rst)
  delay_tree5/4(out4) -> [n4]
  delay_tree5/5(out5) -> [n5]
  Constant2/1 -> Relational2/2
  delay_tree2/3(out3) -> [rst3]
  delay_tree4/1(out1) -> [re1]
  delay_tree3/4(out4) -> [im4]
  [rst1] -> msdft/3(rst)
  [re3] -> msdft1/5(twidd_re)
  [n3] -> Relational2/1
  delay_tree6/2(out2) -> [addr2]
  "sync "/1 -> delay_tree1/1(in)
  [addr5] -> msdft3/7(mem_addr)
  delay_tree/2(out2) -> [din2]
  delay_tree1/2(out2) -> [sync2]
  twidd_re/1 -> delay_tree4/1(in)
  delay_tree/3(out3) -> [din3]
  [din2] -> msdft4/1(din)
  Relational4/1 -> msdft3/6(we_twidd)
  [re5] -> msdft3/5(twidd_re)
  Relational1/1 -> msdft4/6(we_twidd)
  [re4] -> msdft2/5(twidd_re)
  delay_tree2/5(out5) -> [rst5]
  [sync4] -> msdft2/2(sync)
  delay_tree2/2(out2) -> [rst2]
  delay_tree/1(out1) -> [din1]
  [re2] -> msdft4/5(twidd_re)
  [sync1] -> Delay/1, msdft/2(sync)
  delay_tree4/3(out3) -> [re3]
  din/1 -> delay_tree/1(in)
  [sync5] -> msdft3/2(sync)
  [din4] -> msdft2/1(din)
  delay_tree3/1(out1) -> [im1]
  delay_tree1/4(out4) -> [sync4]
  delay_tree4/2(out2) -> [re2]
  [n5] -> Relational4/1
  delay_tree5/2(out2) -> [n2]
  [sync3] -> msdft1/2(sync)
  delay_tree1/5(out5) -> [sync5]
  delay_tree5/3(out3) -> [n3]
  [addr2] -> msdft4/7(mem_addr)
  [rst4] -> msdft2/3(rst)
  twidd_num/1 -> delay_tree5/1(in)
  Constant1/1 -> Relational3/2
  delay_tree5/1(out1) -> [n1]
  [din3] -> msdft1/1(din)
  rst/1 -> delay_tree2/1(in)
  msdft2/1(dout) -> Out4/1
  [addr1] -> msdft/7(mem_addr)
  [addr4] -> msdft2/7(mem_addr)
  delay_tree3/2(out2) -> [im2]
  delay_tree2/1(out1) -> [rst1]
  [im5] -> msdft3/4(twidd_im)
  delay_tree6/4(out4) -> [addr4]
  [n4] -> Relational3/1
  twidd_im/1 -> delay_tree3/1(in)
  [im1] -> msdft/4(twidd_im)
  delay_tree3/5(out5) -> [im5]
  msdft/1(dout) -> Out1/1
  [im4] -> msdft2/4(twidd_im)
  Relational/1 -> msdft/6(we_twidd)
  delay_tree3/3(out3) -> [im3]
  delay_tree2/4(out4) -> [rst4]
  [n2] -> Relational1/1
  [din1] -> msdft/1(din)
  delay_tree1/1(out1) -> [sync1]
  [im3] -> msdft1/4(twidd_im)
  Constant/1 -> Relational4/2
  delay_tree4/4(out4) -> [re4]
  [im2] -> msdft4/4(twidd_im)
  delay_tree4/5(out5) -> [re5]
  delay_tree6/5(out5) -> [addr5]
  delay_tree1/3(out3) -> [sync3]
  [rst3] -> msdft1/3(rst)
  [rst2] -> msdft4/3(rst)
  [n1] -> Relational/1
  Relational2/1 -> msdft1/6(we_twidd)
  [sync2] -> msdft4/2(sync)
  [re1] -> msdft/5(twidd_re)
  delay_tree/4(out4) -> [din4]
  Relational3/1 -> msdft2/6(we_twidd)
  mem_addr/1 -> delay_tree6/1(in)
  delay_tree/5(out5) -> [din5]
  Delay/1 -> sync_out/1
  msdft4/1(dout) -> Out2/1
  msdft3/1(dout) -> Out5/1

== system msdft_12_v2/msdft_sel ==
  sim_1 : Inport
  io_delay : xbsIndex_r4/Delay  rst=off  infoeditControl=Selection of Reset will increase slice count due to use of real FFs and instead of SRLs  en=off  latency=0  dbl_ovrd=off  reg_retiming=on  block_type=delay
  msdft_12_v2_msdft_sel_user_data_out : xbsIndex_r4/Gateway In  gui_display_data_type=Fixed-point  arith_type=Unsigned  n_bits=32  bin_pt=0  preci_type=Single  exp_width=8  frac_width=24  quantization="Round  (unbiased: +/- Inf)"  overflow=Saturate  period=1  dbl_ovrd=off  timing_constraint=None  locs_specified=off  LOCs={}  UseAsADC=off  ADCChannel='1'  inherit_from_input=off  hdl_port=on  block_type=gatewayin
  reint1 : xbsIndex_r4/Reinterpret  force_arith_type=on  arith_type=Unsigned  force_bin_pt=on  bin_pt=0  block_type=reinterpret
  slice_reg : xbsIndex_r4/Slice  nbits=32  boolean_output=off  mode=Lower Bit Location + Width  bit1=0  base1=MSB of Input  bit0=0  base0=LSB of Input  dbl_ovrd=off  block_type=slice
  in_reg : Outport
  wires:
  msdft_12_v2_msdft_sel_user_data_out/1 -> io_delay/1
  sim_1/1 -> msdft_12_v2_msdft_sel_user_data_out/1
  io_delay/1 -> slice_reg/1
  slice_reg/1 -> reint1/1
  reint1/1 -> in_reg/1

== system msdft_12_v2/rst ==
  sim_1 : Inport
  io_delay : xbsIndex_r4/Delay  rst=off  infoeditControl=Selection of Reset will increase slice count due to use of real FFs and instead of SRLs  en=off  latency=0  dbl_ovrd=off  reg_retiming=on  block_type=delay
  msdft_12_v2_rst_user_data_out : xbsIndex_r4/Gateway In  gui_display_data_type=Fixed-point  arith_type=Unsigned  n_bits=32  bin_pt=0  preci_type=Single  exp_width=8  frac_width=24  quantization="Round  (unbiased: +/- Inf)"  overflow=Saturate  period=1  dbl_ovrd=off  timing_constraint=None  locs_specified=off  LOCs={}  UseAsADC=off  ADCChannel='1'  inherit_from_input=off  hdl_port=on  block_type=gatewayin
  slice_reg : xbsIndex_r4/Slice  nbits=32  boolean_output=on  mode=Lower Bit Location + Width  bit1=0  base1=MSB of Input  bit0=0  base0=LSB of Input  dbl_ovrd=off  block_type=slice
  in_reg : Outport
  wires:
  msdft_12_v2_rst_user_data_out/1 -> io_delay/1
  sim_1/1 -> msdft_12_v2_rst_user_data_out/1
  io_delay/1 -> slice_reg/1
  slice_reg/1 -> in_reg/1

== system msdft_12_v2/rst_cycles ==
  sim_1 : Inport
  io_delay : xbsIndex_r4/Delay  rst=off  infoeditControl=Selection of Reset will increase slice count due to use of real FFs and instead of SRLs  en=off  latency=0  dbl_ovrd=off  reg_retiming=on  block_type=delay
  msdft_12_v2_rst_cycles_user_data_out : xbsIndex_r4/Gateway In  gui_display_data_type=Fixed-point  arith_type=Unsigned  n_bits=32  bin_pt=0  preci_type=Single  exp_width=8  frac_width=24  quantization="Round  (unbiased: +/- Inf)"  overflow=Saturate  period=1  dbl_ovrd=off  timing_constraint=None  locs_specified=off  LOCs={}  UseAsADC=off  ADCChannel='1'  inherit_from_input=off  hdl_port=on  block_type=gatewayin
  reint1 : xbsIndex_r4/Reinterpret  force_arith_type=on  arith_type=Unsigned  force_bin_pt=on  bin_pt=0  block_type=reinterpret
  slice_reg : xbsIndex_r4/Slice  nbits=32  boolean_output=off  mode=Lower Bit Location + Width  bit1=0  base1=MSB of Input  bit0=0  base0=LSB of Input  dbl_ovrd=off  block_type=slice
  in_reg : Outport
  wires:
  msdft_12_v2_rst_cycles_user_data_out/1 -> io_delay/1
  sim_1/1 -> msdft_12_v2_rst_cycles_user_data_out/1
  io_delay/1 -> slice_reg/1
  slice_reg/1 -> reint1/1
  reint1/1 -> in_reg/1

== system msdft_12_v2/rst_save ==
  sim_1 : Inport
  io_delay : xbsIndex_r4/Delay  rst=off  infoeditControl=Selection of Reset will increase slice count due to use of real FFs and instead of SRLs  en=off  latency=0  dbl_ovrd=off  reg_retiming=on  block_type=delay
  msdft_12_v2_rst_save_user_data_out : xbsIndex_r4/Gateway In  gui_display_data_type=Fixed-point  arith_type=Unsigned  n_bits=32  bin_pt=0  preci_type=Single  exp_width=8  frac_width=24  quantization="Round  (unbiased: +/- Inf)"  overflow=Saturate  period=1  dbl_ovrd=off  timing_constraint=None  locs_specified=off  LOCs={}  UseAsADC=off  ADCChannel='1'  inherit_from_input=off  hdl_port=on  block_type=gatewayin
  slice_reg : xbsIndex_r4/Slice  nbits=32  boolean_output=on  mode=Lower Bit Location + Width  bit1=0  base1=MSB of Input  bit0=0  base0=LSB of Input  dbl_ovrd=off  block_type=slice
  in_reg : Outport
  wires:
  msdft_12_v2_rst_save_user_data_out/1 -> io_delay/1
  sim_1/1 -> msdft_12_v2_rst_save_user_data_out/1
  io_delay/1 -> slice_reg/1
  slice_reg/1 -> in_reg/1
